simulink model "STModel_with_MMAE"  (R2018b)
settings: Solver=FixedStepDiscrete  StartTime=0.0  StopTime=6  FixedStep=Tsmall  RelTol=1e-3  EnableMultiTasking=on
PreLoadFcn:
  | if exist('tl_preloadfcn','file'), tl_preloadfcn(gcs,403); end
PostLoadFcn:
  | if exist('tl_postloadfcn','file'), tl_postloadfcn(gcs,403); end
InitFcn:
  | if exist('tlds_init','file'), tlds_init(gcs); end
StartFcn:
  | if exist('tlds_start','file'), tlds_start(gcs); end
StopFcn:
  | if exist('tlds_stop','file'), tlds_stop(gcs); end
values from neighbouring files (symbols this model uses):
  l = obj.vehicleParameters.l_r + obj.vehicleParameters.l_f    [SimplifiedKinematicBicycleModel.m]
  l_r = obj.vehicleParameters.l_r    [KinematicBicycleModel.m]
  Ts = 0.1    [KinematicBicycleModel.m]    (also in LeftLaneChangeSinusoidalMotionModel.m; LinearizedBicycleModel.m; SimplifiedKinematicBicycleModel.m; amm_rel_test.m)
  Ts_bp = 0.01    [initialization.m]    (also in laneChangeSinusoidalFcn.m; laneChangeSinusoidalJacobianFcn.m; leftLaneChangeParametricFcn.m; leftLaneChangeParametricWithAccFcn.m)
  vx = X(2)    [cv_model_fun.m]    (also in initialization.m = 10)
  vy = X(4)    [cv_model_fun.m]    (also in initialization.m = 0)
  x = X(1)    [KinematicBicycleModel.m]    (also in SimplifiedKinematicBicycleModel.m; behavior_model.m = 0:0.01:20; cca_model_fun.m; ctra_model_fun.m)
  y = X(2)    [KinematicBicycleModel.m]    (also in SimplifiedKinematicBicycleModel.m; behavior_model.m = [distances velocities]; cca_model_fun.m; ctra_model_fun.m)
undefined symbols (not defined in the file or in its folder): alpha_f0, alpha_r0, Bm1, Bsc, Bx_ash_f, Bx_ash_r, Bx_snow_f, Bx_snow_r, Bx_wash_f, Bx_wash_r, By_ash_f, By_ash_r, By_snow_f, By_snow_r, By_wash_f, By_wash_r, Cx_ash_f, Cx_ash_r, Cx_snow_f, Cx_snow_r, Cx_wash_f, Cx_wash_r, Cy_ash_f, Cy_ash_r, Cy_snow_f, Cy_snow_r, Cy_wash_f, Cy_wash_r, Ex_ash_f, Ex_ash_r, Ex_snow_f, Ex_snow_r, Ex_wash_f, Ex_wash_r, Ey_ash_f, Ey_ash_r, Ey_snow_f, Ey_snow_r, Ey_wash_f, Ey_wash_r, g, Im1, Isw, Iw, Iz, Kb1, Ks1, kt1, l_f, m, mu_x_ash_f, mu_x_ash_r, mu_x_snow_f, mu_x_snow_r, mu_x_wash_f, mu_x_wash_r, mu_y_ash_f, mu_y_ash_r, mu_y_snow_f, mu_y_snow_r ... (+18)
libraries: simulink x6
(part 1 of 2)
PreSaveFcn:
  | if exist('tl_presavefcn','file'), tl_presavefcn(gcs); end
CloseFcn:
  | if exist('tl_closefcn','file'), tl_closefcn(gcs); end
settings Model: TLRevision=403  ExtModeTrigDuration=10000  Creator=srivats  LastModifiedBy=jasprit
settings SolverCC: PositivePriorityOrder=on  AutoInsertRateTranBlk=on
settings DebuggingCC: LibraryContextMissingDiagnostic=none
settings SFSimCC: SimUseLocalCustomCode=off
settings RTWCC: SystemTargetFile=quarc_win64.tlc  TemplateMakefile=quarc_default_tmf  Description=QUARC Win64 Target  RTWUseLocalCustomCode=off
settings STFCustomTargetCC: TargetPreCompLibLocation=C:\PROGRA~3\QUARC\lib\2018a\win64\release  TargetLangStandard=C99 (ISO)  ConcurrentExecutionCompliant=on  GRTInterface=on  SystemTargetFile=quarc_win64.tlc
settings GRTTargetCC: TargetPreCompLibLocation=C:\PROGRA~3\QUARC\lib\2018a\win64\release  ParMdlRefBuildCompliant=off  CompOptLevelCompliant=off  CombineOutputUpdateFcns=off  MatFileLogging=off  CPPClassGenCompliant=off  GRTInterface=on  UseToolchainInfoCompliant=off  ExtMode=on  ExtModeMexFile=quarc_comm

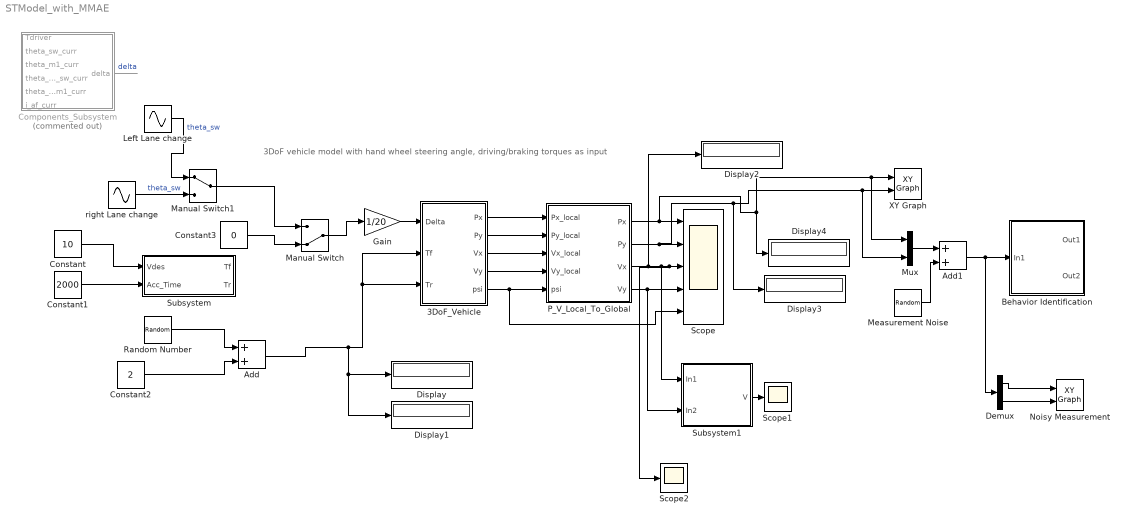
== system STModel_with_MMAE ==
  note: 3DoF vehicle model with hand wheel steering angle, driving/braking torques as input
  3DoF_Vehicle : Subsystem
  Add : Sum
  Add1 : Sum
  Behavior Identification : Subsystem
  Components_Subsystem : Subsystem  Commented=on
  Constant : Constant  Value=10
  Constant1 : Constant  Value=2000
  Constant2 : Constant  Value=2
  Constant3 : Constant  Value=0
  Demux : Demux  Outputs=2
  Display{,1..4} (5 alike) : Display
  Gain : Gain  Gain=1/20
  Left Lane change : Sin  Amplitude=0.11  Frequency=2*pi/10  SampleTime=0.001
  Manual Switch : ManualSwitch  CurrentSetting=0
  Manual Switch1 : ManualSwitch
  "Measurement Noise " : RandomNumber  Variance=0.025
  Mux : Mux  Inputs=2
  Noisy Measurement : simulink/Sinks/XY Graph  xmin=-10  xmax=100  ymin=-5  ymax=5  st=-1
  P_V_Local_To_Global : Subsystem
  Random Number : RandomNumber  SampleTime=0.001
  Scope : Scope  NumInputPorts=5
  Scope1 : Scope
  Scope2 : Scope
  Subsystem : Subsystem
  Subsystem1 : Subsystem
  XY Graph : simulink/Sinks/XY Graph  xmin=-10  xmax=100  ymin=-5  ymax=5  st=-1
  right Lane change : Sin  Amplitude=0.11  Frequency=2*pi/10  Phase=-pi  SampleTime=0.001
  wires:
  Components_Subsystem/1(delta) -> ?  "delta"
  3DoF_Vehicle/1(Px) -> P_V_Local_To_Global/1(Px_local)
  3DoF_Vehicle/2(Py) -> P_V_Local_To_Global/2(Py_local)
  3DoF_Vehicle/4(Vy) -> P_V_Local_To_Global/4(Vy_local)
  3DoF_Vehicle/5(psi) -> Scope/5, P_V_Local_To_Global/5(psi)
  P_V_Local_To_Global/1(Px) -> Display4/1, Mux/1, XY Graph/1, Scope/1
  P_V_Local_To_Global/2(Py) -> Display3/1, Mux/2, XY Graph/2, Scope/2
  P_V_Local_To_Global/3(Vx) -> Display2/1, Subsystem1/1(In1), Scope2/1, Scope/3
  P_V_Local_To_Global/4(Vy) -> Subsystem1/2(In2), Scope/4
  Gain/1 -> 3DoF_Vehicle/1(Delta)
  Left Lane change/1 -> Manual Switch1/1  "theta_sw"
  Constant/1 -> Subsystem/1(Vdes)
  Constant1/1 -> Subsystem/2(Acc_Time)
  Subsystem1/1(V) -> Scope1/1
  3DoF_Vehicle/3(Vx) -> P_V_Local_To_Global/3(Vx_local)
  Constant2/1 -> Add/2
  Add/1 -> Display1/1, Display/1, 3DoF_Vehicle/3(Tr), 3DoF_Vehicle/2(Tf)
  Random Number/1 -> Add/1
  Mux/1 -> Add1/1
  "Measurement Noise "/1 -> Add1/2
  Add1/1 -> Demux/1, Behavior Identification/1(In1)
  Demux/1 -> Noisy Measurement/1
  Demux/2 -> Noisy Measurement/2
  Constant3/1 -> Manual Switch/2
  Manual Switch/1 -> Gain/1
  Manual Switch1/1 -> Manual Switch/1
  right Lane change/1 -> Manual Switch1/2  "theta_sw"

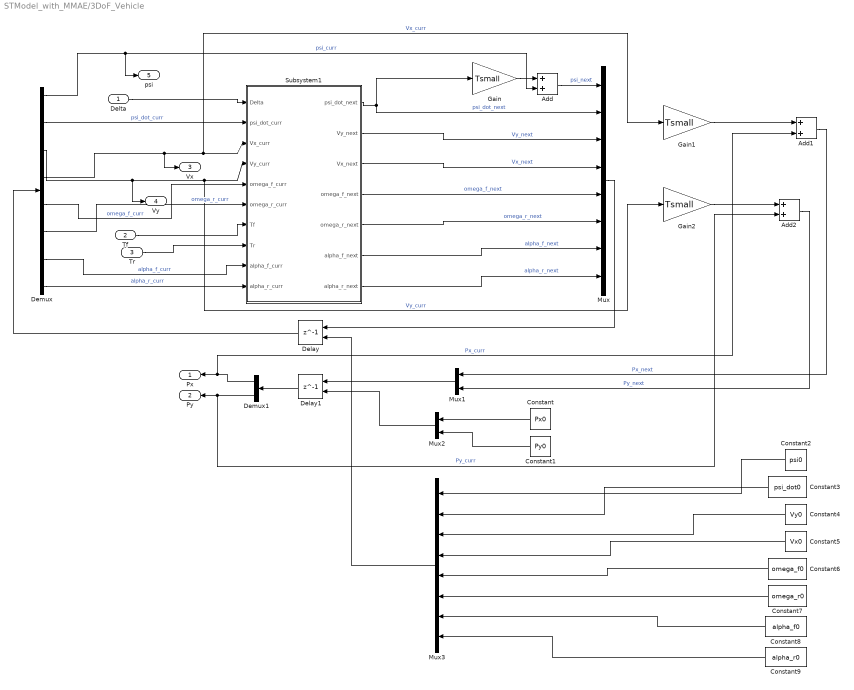
== system STModel_with_MMAE/3DoF_Vehicle ==
  Delta : Inport
  Tf : Inport  Port=2
  Tr : Inport  Port=3
  Add : Sum
  Add1 : Sum
  Add2 : Sum
  Constant : Constant  Value=Px0
  Constant1 : Constant  Value=Py0
  Constant2 : Constant  Value=psi0
  Constant3 : Constant  Value=psi_dot0
  Constant4 : Constant  Value=Vy0
  Constant5 : Constant  Value=Vx0
  Constant6 : Constant  Value=omega_f0
  Constant7 : Constant  Value=omega_r0
  Constant8 : Constant  Value=alpha_f0
  Constant9 : Constant  Value=alpha_r0
  Delay : Delay  DelayLength=1  InitialConditionSource=Input port  SampleTime=Tsmall
      settings: InputPortMap=u0,p4
  Delay1 : Delay  DelayLength=1  InitialConditionSource=Input port  SampleTime=Tsmall
      settings: InputPortMap=u0,p4
  Demux : Demux  Outputs=8
  Demux1 : Demux  Outputs=2
  Gain : Gain  Gain=Tsmall
  Gain1 : Gain  Gain=Tsmall
  Gain2 : Gain  Gain=Tsmall
  Mux : Mux  Inputs=8
  Mux1 : Mux  Inputs=2
  Mux2 : Mux  Inputs=2
  Mux3 : Mux  Inputs=8
  Subsystem1 : Subsystem
  Px : Outport
  Py : Outport  Port=2
  Vx : Outport  Port=3
  Vy : Outport  Port=4
  psi : Outport  Port=5
  wires:
  Demux/1 -> psi/1, Add/2  "psi_curr"
  Delay/1 -> Demux/1
  Demux/6 -> Subsystem1/6(omega_r_curr)  "omega_r_curr"
  Gain/1 -> Add/1
  Delta/1 -> Subsystem1/1(Delta)
  Subsystem1/4(omega_f_next) -> Mux/5  "omega_f_next"
  Subsystem1/1(psi_dot_next) -> Mux/2, Gain/1  "psi_dot_next"
  Add/1 -> Mux/1  "psi_next"
  Tr/1 -> Subsystem1/8(Tr)
  Tf/1 -> Subsystem1/7(Tf)
  Subsystem1/3(Vx_next) -> Mux/4  "Vx_next"
  Demux/2 -> Subsystem1/2(psi_dot_curr)  "psi_dot_curr"
  Mux/1 -> Delay/1
  Demux/4 -> Vx/1, Gain1/1, Subsystem1/3(Vx_curr)  "Vx_curr"
  Demux/3 -> Gain2/1, Subsystem1/4(Vy_curr), Vy/1  "Vy_curr"
  Demux/5 -> Subsystem1/5(omega_f_curr)  "omega_f_curr"
  Subsystem1/2(Vy_next) -> Mux/3  "Vy_next"
  Subsystem1/5(omega_r_next) -> Mux/6  "omega_r_next"
  Gain1/1 -> Add1/1
  Gain2/1 -> Add2/1
  Mux1/1 -> Delay1/1
  Add1/1 -> Mux1/1  "Px_next"
  Add2/1 -> Mux1/2  "Py_next"
  Mux2/1 -> Delay1/2
  Constant/1 -> Mux2/1
  Constant1/1 -> Mux2/2
  Delay1/1 -> Demux1/1
  Demux1/1 -> Add1/2, Px/1  "Px_curr"
  Demux1/2 -> Add2/2, Py/1  "Py_curr"
  Constant7/1 -> Mux3/6
  Constant6/1 -> Mux3/5
  Constant3/1 -> Mux3/2
  Constant5/1 -> Mux3/4
  Constant4/1 -> Mux3/3
  Constant2/1 -> Mux3/1
  Mux3/1 -> Delay/2
  Subsystem1/6(alpha_f_next) -> Mux/7  "alpha_f_next"
  Subsystem1/7(alpha_r_next) -> Mux/8  "alpha_r_next"
  Constant8/1 -> Mux3/7
  Constant9/1 -> Mux3/8
  Demux/7 -> Subsystem1/9(alpha_f_curr)  "alpha_f_curr"
  Demux/8 -> Subsystem1/10(alpha_r_curr)  "alpha_r_curr"

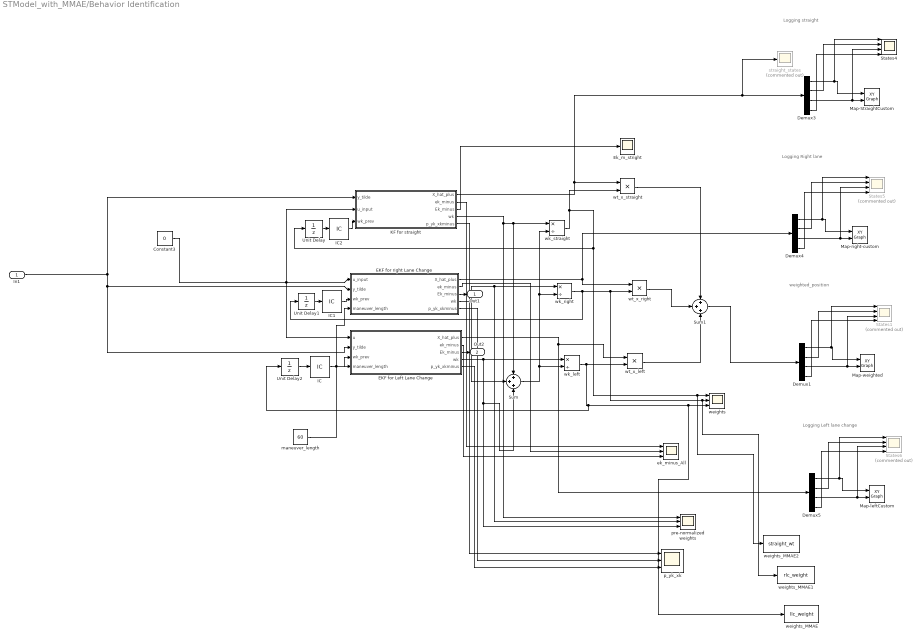
== system STModel_with_MMAE/Behavior Identification ==
  note: weighted_position
  note: Logging Right lane
  note: Logging straight
  note: Logging Left lane change
  In1 : Inport  SampleTime=Ts_bp
  Constant3 : Constant  Value=0
  Demux{1,3..5} (4 alike) : Demux
  EKF for Left Lane Change : Subsystem
  EKF for right Lane Change : Subsystem
  Ek_m_stright : Scope
  IC : InitialCondition  Value=1/3
  IC1 : InitialCondition  Value=1/3
  IC2 : InitialCondition  Value=1/3
  KF for straight : Subsystem
  Map-StraightCustom : simulink/Sinks/XY Graph  xmin=-1  xmax=200  ymin=-20  ymax=20  st=-1
  Map-leftCustom : simulink/Sinks/XY Graph  xmin=-1  xmax=300  ymin=-5  ymax=5  st=-1
  Map-right-custom : simulink/Sinks/XY Graph  xmin=-1  xmax=300  ymin=-5  ymax=5  st=-1
  Map-weighted : simulink/Sinks/XY Graph  xmin=-1  xmax=300  ymin=-5  ymax=5  st=-1
  States1 : Scope  Commented=on  NumInputPorts=4
  States4 : Scope  NumInputPorts=4
  States5 : Scope  Commented=on  NumInputPorts=4
  States6 : Scope  Commented=on  NumInputPorts=4
  Sum : Sum  Inputs=+++
  Sum1 : Sum  Inputs=+++
  Unit Delay : UnitDelay  SampleTime=Ts_bp
  Unit Delay1 : UnitDelay  SampleTime=Ts_bp
  Unit Delay2 : UnitDelay  SampleTime=Ts_bp
  ek_minus_All : Scope  NumInputPorts=3
  maneuver_length : Constant  Value=60
  p_yk_xk : Scope  NumInputPorts=3
  pre-normalized weights : Scope  NumInputPorts=3
  straight_states : Scope  Commented=on
  weights : Scope  NumInputPorts=3
  weights_MMAE : ToWorkspace  VariableName=llc_weight  SaveFormat=Structure With Time  SampleTime=-1
  weights_MMAE1 : ToWorkspace  VariableName=rlc_weight  SaveFormat=Structure With Time  SampleTime=-1
  weights_MMAE2 : ToWorkspace  VariableName=straight_wt  SaveFormat=Structure With Time  SampleTime=-1
  wk_left : Product  Inputs=*/
  wk_right : Product  Inputs=*/
  wk_straight : Product  Inputs=*/
  wt_x_left : Product  Inputs=**
  wt_x_right : Product  Inputs=**
  wt_x_straight : Product  Inputs=**
  Out1 : Outport
  Out2 : Outport  Port=2
  wires:
  Demux3/4 -> States4/4
  Demux1/2 -> States1/2
  EKF for Left Lane Change/2(ek_minus) -> ek_minus_All/3
  EKF for right Lane Change/1(X_hat_plus) -> Demux4/1, wt_x_right/1
  KF for straight/1(X_hat_plus) -> straight_states/1, Demux3/1, wt_x_straight/1
  In1/1 -> EKF for Left Lane Change/2(y_tilde), EKF for right Lane Change/2(y_tilde), KF for straight/1(y_tilde)
  wk_straight/1 -> Unit Delay/1, weights/1, weights_MMAE2/1, wt_x_straight/2
  wt_x_right/1 -> Sum1/2
  Demux4/3 -> Map-right-custom/2, States5/3
  EKF for Left Lane Change/1(X_hat_plus) -> wt_x_left/1, Demux5/1
  wk_left/1 -> Unit Delay2/1, weights_MMAE/1, weights/3, wt_x_left/2
  Demux5/1 -> States6/1, Map-leftCustom/1
  EKF for Left Lane Change/3(Ek_minus) -> Out2/1
  IC1/1 -> EKF for right Lane Change/3(wk_prev)
  maneuver_length/1 -> EKF for right Lane Change/4(maneuver_length), EKF for Left Lane Change/4(maneuver_length)
  EKF for right Lane Change/3(Ek_minus) -> Out1/1
  Demux1/1 -> States1/1, Map-weighted/1
  KF for straight/4(wk) -> pre-normalized weights/1, wk_straight/1, Sum/1
  KF for straight/5(p_yk_xkminus) -> p_yk_xk/1
  EKF for Left Lane Change/4(wk) -> wk_left/1, pre-normalized weights/3, Sum/3
  Sum/1 -> wk_left/2, wk_straight/2, wk_right/2
  Demux4/1 -> States5/1, Map-right-custom/1
  Demux1/4 -> States1/4
  Demux3/1 -> States4/1, Map-StraightCustom/1
  Constant3/1 -> KF for straight/2(u_input), EKF for right Lane Change/1(u_input), EKF for Left Lane Change/1(u)
  wk_right/1 -> Unit Delay1/1, weights_MMAE1/1, weights/2, wt_x_right/2
  Unit Delay/1 -> IC2/1
  wt_x_straight/1 -> Sum1/1
  EKF for right Lane Change/2(ek_minus) -> ek_minus_All/2
  Demux5/2 -> States6/2
  Demux5/3 -> Map-leftCustom/2, States6/3
  wt_x_left/1 -> Sum1/3
  Unit Delay2/1 -> IC/1
  Demux1/3 -> States1/3, Map-weighted/2
  KF for straight/2(ek_minus) -> ek_minus_All/1
  EKF for right Lane Change/4(wk) -> pre-normalized weights/2, wk_right/1, Sum/2
  EKF for Left Lane Change/5(p_yk_xkminus) -> p_yk_xk/3
  Demux5/4 -> States6/4
  Sum1/1 -> Demux1/1
  Unit Delay1/1 -> IC1/1
  Demux4/4 -> States5/4
  Demux3/3 -> Map-StraightCustom/2, States4/3
  EKF for right Lane Change/5(p_yk_xkminus) -> p_yk_xk/2
  IC/1 -> EKF for Left Lane Change/3(wk_prev)
  IC2/1 -> KF for straight/3(wk_prev)
  KF for straight/3(Ek_minus) -> Ek_m_stright/1
  Demux3/2 -> States4/2
  Demux4/2 -> States5/2

== system STModel_with_MMAE/Components_Subsystem ==
  Tdriver : Inport
  theta_sw_curr : Inport  Port=2
  theta_m1_curr : Inport  Port=3
  theta_dot_sw_curr : Inport  Port=4
  theta_dot_m1_curr : Inport  Port=5
  i_af_curr : Inport  Port=6
  Euler_Integrator1 : Subsystem
  Euler_Integrator2 : Subsystem
  Euler_Integrator3 : Subsystem
  Euler_Integrator4 : Subsystem
  Euler_Integrator5 : Subsystem
  Gain : Gain  Gain=kt1
  Subsystem : Subsystem
  Theta_M1_Subsystem : Subsystem
  Theta_SW_Subsystem : Subsystem
  delta : Outport
  wires:
  Tdriver/1 -> Theta_SW_Subsystem/1(Tdriver)
  theta_dot_sw_curr/1 -> Euler_Integrator1/1(state_dot), Euler_Integrator2/2(state_curr), Theta_SW_Subsystem/2(theta_dot_sw)
  theta_dot_m1_curr/1 -> Euler_Integrator4/1(state_dot), Euler_Integrator3/2(state_curr), Theta_SW_Subsystem/3(theta_dot_m1)  "theta_dot_m1"
  theta_sw_curr/1 -> Euler_Integrator1/2(state_curr), Theta_SW_Subsystem/4(theta_sw)
  theta_m1_curr/1 -> Euler_Integrator4/2(state_curr), Theta_SW_Subsystem/5(theta_m1)  "theta_m1_curr"
  Theta_SW_Subsystem/1(theta_sw_ddot) -> Euler_Integrator2/1(state_dot)
  Euler_Integrator2/1(state_next) -> ?  "theta_sw_dot_next"
  Euler_Integrator1/1(state_next) -> ?  "theta_sw_curr"
  Theta_M1_Subsystem/1("theta_m1_ddot ") -> Euler_Integrator3/1(state_dot)
  Euler_Integrator3/1(state_next) -> ?  "theta_m1_dot_next"
  Euler_Integrator4/1(state_next) -> ?  "theta_m1_next"
  i_af_curr/1 -> Gain/1, Euler_Integrator5/2(state_curr), Subsystem/1(i_a1)  "i_af"
  Subsystem/1(i_a1_dot) -> Euler_Integrator5/1(state_dot)
  Euler_Integrator5/1(state_next) -> ?  "i_af_next"
  Gain/1 -> Theta_M1_Subsystem/5(Tm1)

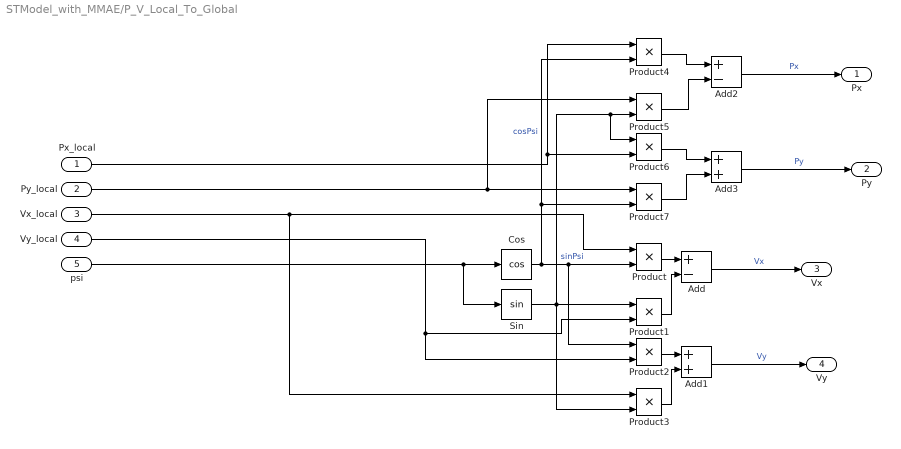
== system STModel_with_MMAE/P_V_Local_To_Global ==
  Px_local : Inport  OutDataTypeStr=double  SampleTime=Ts
  Py_local : Inport  Port=2  OutDataTypeStr=double  SampleTime=Ts
  Vx_local : Inport  Port=3  OutDataTypeStr=double  SampleTime=Ts
  Vy_local : Inport  Port=4  OutDataTypeStr=double  SampleTime=Ts
  psi : Inport  Port=5  OutDataTypeStr=double  SampleTime=Ts
  Add : Sum  Inputs=+-
  Add1 : Sum
  Add2 : Sum  Inputs=+-
  Add3 : Sum
  Cos : Trigonometry  Operator=cos
  Product{,1..7} (8 alike) : Product
  Sin : Trigonometry
  Px : Outport  OutDataTypeStr=double  SampleTime=Ts
  Py : Outport  Port=2  OutDataTypeStr=double  SampleTime=Ts
  Vx : Outport  Port=3  OutDataTypeStr=double  SampleTime=Ts
  Vy : Outport  Port=4  OutDataTypeStr=double  SampleTime=Ts
  wires:
  Px_local/1 -> Product4/1, Product6/2
  Py_local/1 -> Product7/1, Product5/1
  Vx_local/1 -> Product3/1, Product/1
  Product5/1 -> Add2/2
  Product4/1 -> Add2/1
  Add2/1 -> Px/1  "Px"
  Product7/1 -> Add3/2
  Sin/1 -> Product6/1, Product5/2, Product3/2, Product1/1  "sinPsi"
  Vy_local/1 -> Product1/2, Product2/2
  psi/1 -> Sin/1, Cos/1
  Cos/1 -> Product7/2, Product4/2, Product2/1, Product/2  "cosPsi"
  Add3/1 -> Py/1  "Py"
  Product2/1 -> Add1/1
  Product1/1 -> Add/2
  Add/1 -> Vx/1  "Vx"
  Add1/1 -> Vy/1  "Vy"
  Product6/1 -> Add3/1
  Product3/1 -> Add1/2
  Product/1 -> Add/1

== system STModel_with_MMAE/Subsystem ==
  Vdes : Inport
  Acc_Time : Inport  Port=2
  Add : Sum
  Constant : Constant  Value=RR
  Divide : Product  Inputs=*/
  Gain : Gain  Gain=9.81
  Gain1 : Gain  Gain=m
  Gain2 : Gain  Gain=0.5
  Tf : Outport
  Tr : Outport  Port=2
  wires:
  Vdes/1 -> Gain1/1
  Acc_Time/1 -> Gain/1
  Gain1/1 -> Divide/1
  Gain/1 -> Divide/2
  Divide/1 -> Add/1  "Fa"
  Constant/1 -> Add/2
  Add/1 -> Gain2/1  "TTE"
  Gain2/1 -> Tf/1, Tr/1

== system STModel_with_MMAE/Subsystem1 ==
  In1 : Inport
  In2 : Inport  Port=2
  Add : Sum
  Sqrt : Sqrt  SaturateOnIntegerOverflow=on
  Square : Math  Operator=square  SaturateOnIntegerOverflow=on
  Square1 : Math  Operator=square  SaturateOnIntegerOverflow=on
  V : Outport
  wires:
  Square1/1 -> Add/2
  In1/1 -> Square/1
  Add/1 -> Sqrt/1
  Square/1 -> Add/1
  Sqrt/1 -> V/1  "V"
  In2/1 -> Square1/1

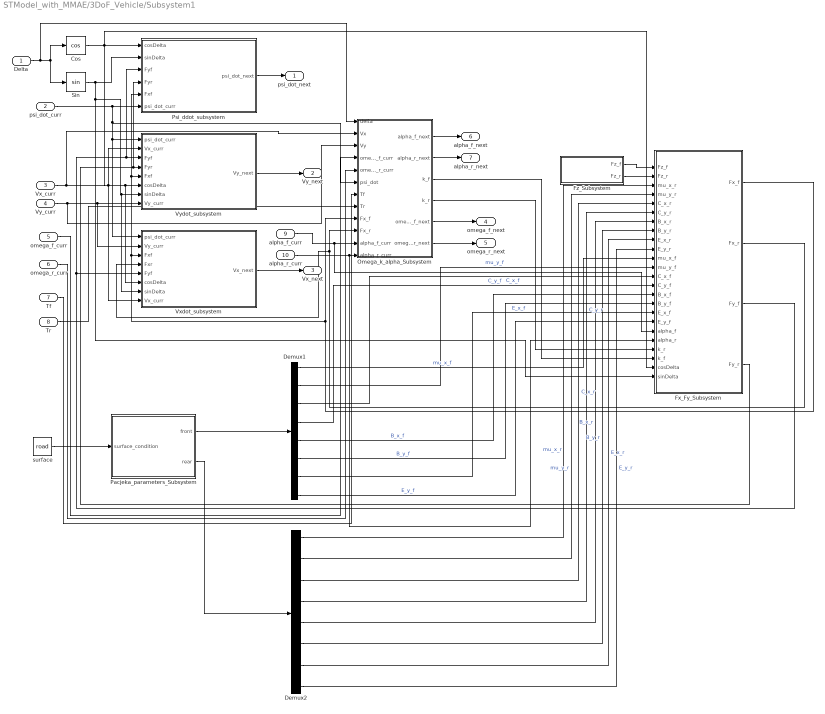
== system STModel_with_MMAE/3DoF_Vehicle/Subsystem1 ==
  Delta : Inport
  psi_dot_curr : Inport  Port=2
  Vx_curr : Inport  Port=3
  Vy_curr : Inport  Port=4
  omega_f_curr : Inport  Port=5
  omega_r_curr : Inport  Port=6
  Tf : Inport  Port=7
  Tr : Inport  Port=8
  alpha_f_curr : Inport  Port=9
  alpha_r_curr : Inport  Port=10
  Cos : Trigonometry  Operator=cos
  Demux1 : Demux  Outputs=8
  Demux2 : Demux  Outputs=8
  Fx_Fy_Subsystem : Subsystem
  Fz_Subsystem : Subsystem
  Omega_k_alpha_Subsystem : Subsystem
  Pacjeka_parameters_Subsystem : Subsystem
  Psi_ddot_subsystem : Subsystem
  Sin : Trigonometry
  Vxdot_subsystem : Subsystem
  Vydot_subsystem : Subsystem
  surface : Constant  Value=road
  psi_dot_next : Outport
  Vy_next : Outport  Port=2
  Vx_next : Outport  Port=3
  omega_f_next : Outport  Port=4
  omega_r_next : Outport  Port=5
  alpha_f_next : Outport  Port=6
  alpha_r_next : Outport  Port=7
  wires:
  Omega_k_alpha_Subsystem/4(k_r) -> Fx_Fy_Subsystem/21(k_r)
  Fx_Fy_Subsystem/2(Fx_r) -> Vxdot_subsystem/4(Fxr), Omega_k_alpha_Subsystem/10(Fx_r)
  Fx_Fy_Subsystem/1(Fx_f) -> Omega_k_alpha_Subsystem/9(Fx_f), Vxdot_subsystem/3(Fxf), Psi_ddot_subsystem/5(Fxf), Vydot_subsystem/5(Fxf)
  Omega_k_alpha_Subsystem/3(k_f) -> Fx_Fy_Subsystem/22(k_f)
  Sin/1 -> Fx_Fy_Subsystem/24(sinDelta), Vxdot_subsystem/7(sinDelta), Vydot_subsystem/7(sinDelta), Psi_ddot_subsystem/2(sinDelta)
  Vydot_subsystem/1(Vy_next) -> Vy_next/1
  Fx_Fy_Subsystem/3(Fy_f) -> Psi_ddot_subsystem/3(Fyf), Vydot_subsystem/3(Fyf), Vxdot_subsystem/5(Fyf)
  psi_dot_curr/1 -> Omega_k_alpha_Subsystem/6(psi_dot), Vydot_subsystem/1(psi_dot_curr), Vxdot_subsystem/1(psi_dot_curr), Psi_ddot_subsystem/6(psi_dot_curr)
  Fx_Fy_Subsystem/4(Fy_r) -> Psi_ddot_subsystem/4(Fyr), Vydot_subsystem/4(Fyr)
  Cos/1 -> Fx_Fy_Subsystem/23(cosDelta), Vxdot_subsystem/6(cosDelta), Vydot_subsystem/6(cosDelta), Psi_ddot_subsystem/1(cosDelta)
  Tf/1 -> Omega_k_alpha_Subsystem/7(Tf)
  Demux1/7 -> Fx_Fy_Subsystem/17(E_x_f)  "E_x_f"
  omega_f_curr/1 -> Omega_k_alpha_Subsystem/4(omega_f_curr)
  Vy_curr/1 -> Omega_k_alpha_Subsystem/3(Vy), Vxdot_subsystem/2(Vy_curr), Vydot_subsystem/8(Vy_curr)
  Pacjeka_parameters_Subsystem/1(front) -> Demux1/1
  Omega_k_alpha_Subsystem/6(omega_r_next) -> omega_r_next/1
  Delta/1 -> Omega_k_alpha_Subsystem/1(delta), Sin/1, Cos/1
  Vx_curr/1 -> Omega_k_alpha_Subsystem/2(Vx), Vydot_subsystem/2(Vx_curr), Vxdot_subsystem/8(Vx_curr)
  Demux1/1 -> Fx_Fy_Subsystem/11(mu_x_f)  "mu_x_f"
  Vxdot_subsystem/1(Vx_next) -> Vx_next/1
  Omega_k_alpha_Subsystem/5(omega_f_next) -> omega_f_next/1
  Demux2/4 -> Fx_Fy_Subsystem/6(C_y_r)  "C_y_r"
  Fz_Subsystem/1(Fz_f) -> Fx_Fy_Subsystem/1(Fz_f)
  Tr/1 -> Omega_k_alpha_Subsystem/8(Tr)
  omega_r_curr/1 -> Omega_k_alpha_Subsystem/5(omega_r_curr)
  surface/1 -> Pacjeka_parameters_Subsystem/1(surface_condition)
  Pacjeka_parameters_Subsystem/2(rear) -> Demux2/1
  Demux2/7 -> Fx_Fy_Subsystem/9(E_x_r)  "E_x_r"
  Fz_Subsystem/2(Fz_r) -> Fx_Fy_Subsystem/2(Fz_r)
  Demux1/6 -> Fx_Fy_Subsystem/16(B_y_f)  "B_y_f"
  Demux2/6 -> Fx_Fy_Subsystem/8(B_y_r)  "B_y_r"
  Demux2/2 -> Fx_Fy_Subsystem/4(mu_y_r)  "mu_y_r"
  Demux1/8 -> Fx_Fy_Subsystem/18(E_y_f)  "E_y_f"
  Demux2/5 -> Fx_Fy_Subsystem/7(B_x_r)  "B_x_r"
  Psi_ddot_subsystem/1(psi_dot_next) -> psi_dot_next/1
  Demux2/8 -> Fx_Fy_Subsystem/10(E_y_r)  "E_y_r"
  Demux2/1 -> Fx_Fy_Subsystem/3(mu_x_r)  "mu_x_r"
  Demux1/3 -> Fx_Fy_Subsystem/13(C_x_f)  "C_x_f"
  Demux1/4 -> Fx_Fy_Subsystem/14(C_y_f)  "C_y_f"
  Demux1/2 -> Fx_Fy_Subsystem/12(mu_y_f)  "mu_y_f"
  Demux1/5 -> Fx_Fy_Subsystem/15(B_x_f)  "B_x_f"
  Demux2/3 -> Fx_Fy_Subsystem/5(C_x_r)  "C_x_r"
  Omega_k_alpha_Subsystem/1(alpha_f_next) -> alpha_f_next/1
  Omega_k_alpha_Subsystem/2(alpha_r_next) -> alpha_r_next/1
  alpha_r_curr/1 -> Fx_Fy_Subsystem/20(alpha_r), Omega_k_alpha_Subsystem/12(alpha_r_curr)
  alpha_f_curr/1 -> Fx_Fy_Subsystem/19(alpha_f), Omega_k_alpha_Subsystem/11(alpha_f_curr)

== system STModel_with_MMAE/Behavior Identification/EKF for Left Lane Change ==
  u : Inport
  y_tilde : Inport  Port=2
  wk_prev : Inport  Port=3
  maneuver_length : Inport  Port=4
  IC3 : InitialCondition  Value=[x vx y vy]
  MATLAB Function2 : MATLAB Function  TreatAsAtomicUnit=on
  Unit Delay5 : UnitDelay  SampleTime=-1
  Unit Delay6 : UnitDelay  InitialCondition=eye(4)*100  SampleTime=-1
  X_hat_plus : Outport
  ek_minus : Outport  Port=2
  Ek_minus : Outport  Port=3
  wk : Outport  Port=4
  p_yk_xkminus : Outport  Port=5
  wires:
  MATLAB Function2/2(P_plus) -> Unit Delay6/1
  u/1 -> MATLAB Function2/3(u)
  Unit Delay5/1 -> IC3/1
  y_tilde/1 -> MATLAB Function2/4(y_tilde)
  MATLAB Function2/1(X_hat_plus) -> X_hat_plus/1, Unit Delay5/1
  IC3/1 -> MATLAB Function2/1(X)
  Unit Delay6/1 -> MATLAB Function2/2(P)
  MATLAB Function2/3(ek_minus) -> ek_minus/1
  MATLAB Function2/4(ek_m_covariance) -> Ek_minus/1
  MATLAB Function2/5(wk) -> wk/1
  MATLAB Function2/6(p_yk_xkminus) -> p_yk_xkminus/1
  wk_prev/1 -> MATLAB Function2/5(wk_prev)
  maneuver_length/1 -> MATLAB Function2/6(maneuver_length)

== system STModel_with_MMAE/Behavior Identification/EKF for right Lane Change ==
  note: Prior - right lane change
  u_input : Inport
  y_tilde : Inport  Port=2
  wk_prev : Inport  Port=3
  maneuver_length : Inport  Port=4
  IC2 : InitialCondition  Value=[x vx y vy]
  MATLAB Function1 : MATLAB Function  TreatAsAtomicUnit=on
  Unit Delay3 : UnitDelay  InitialCondition=eye(4)*100  SampleTime=-1
  Unit Delay4 : UnitDelay  SampleTime=-1
  X_hat_plus : Outport
  ek_minus : Outport  Port=2
  Ek_minus : Outport  Port=3
  wk : Outport  Port=4
  p_yk_xkminus : Outport  Port=5
  wires:
  MATLAB Function1/2(P_plus) -> Unit Delay3/1
  IC2/1 -> MATLAB Function1/1(X)
  Unit Delay3/1 -> MATLAB Function1/2(P)
  MATLAB Function1/1(X_hat_plus) -> X_hat_plus/1, Unit Delay4/1
  u_input/1 -> MATLAB Function1/3(u)
  y_tilde/1 -> MATLAB Function1/4(y_tilde)
  Unit Delay4/1 -> IC2/1
  MATLAB Function1/3(ek_minus) -> ek_minus/1
  MATLAB Function1/4(ek_m_covariance) -> Ek_minus/1
  wk_prev/1 -> MATLAB Function1/5(wk_prev)
  MATLAB Function1/5(wk) -> wk/1
  MATLAB Function1/6(p_yk_xkminus) -> p_yk_xkminus/1
  maneuver_length/1 -> MATLAB Function1/6(maneuver_length)

== system STModel_with_MMAE/Behavior Identification/KF for straight ==
  note: Prior
  y_tilde : Inport
  u_input : Inport  Port=2
  wk_prev : Inport  Port=3
  IC1 : InitialCondition  Value=[x vx y vy]
  MATLAB Function : MATLAB Function  TreatAsAtomicUnit=on
  Scope : Scope
  Scope1 : Scope
  Unit Delay1 : UnitDelay  SampleTime=-1
  Unit Delay2 : UnitDelay  InitialCondition=eye(4)*100  SampleTime=-1
  X_hat_plus : Outport
  ek_minus : Outport  Port=2
  Ek_minus : Outport  Port=3
  wk : Outport  Port=4
  p_yk_xkminus : Outport  Port=5
  wires:
  Unit Delay2/1 -> MATLAB Function/2(P)
  IC1/1 -> MATLAB Function/1(X)
  MATLAB Function/1(X_hat_plus) -> X_hat_plus/1, Unit Delay1/1
  u_input/1 -> MATLAB Function/3(u)
  Unit Delay1/1 -> IC1/1
  y_tilde/1 -> MATLAB Function/4(y_tilde)
  MATLAB Function/2(P_plus) -> Scope/1, Unit Delay2/1
  MATLAB Function/3(ek_minus) -> ek_minus/1
  MATLAB Function/4(ek_m_covariance) -> Ek_minus/1
  wk_prev/1 -> MATLAB Function/5(wk_prev)
  MATLAB Function/5(wk) -> wk/1
  MATLAB Function/6(p_yk_xkminus) -> p_yk_xkminus/1
  MATLAB Function/7(K) -> Scope1/1

== system STModel_with_MMAE/Components_Subsystem/Euler_Integrator1 ==
  state_dot : Inport
  state_curr : Inport  Port=2
  Add : Sum
  Gain : Gain  Gain=Tsmall
  state_next : Outport
  wires:
  state_dot/1 -> Gain/1
  Gain/1 -> Add/1
  state_curr/1 -> Add/2
  Add/1 -> state_next/1

== system STModel_with_MMAE/Components_Subsystem/Euler_Integrator2 ==
  state_dot : Inport
  state_curr : Inport  Port=2
  Add : Sum
  Gain : Gain  Gain=Tsmall
  state_next : Outport
  wires:
  state_dot/1 -> Gain/1
  Gain/1 -> Add/1
  state_curr/1 -> Add/2
  Add/1 -> state_next/1

== system STModel_with_MMAE/Components_Subsystem/Euler_Integrator3 ==
  state_dot : Inport
  state_curr : Inport  Port=2
  Add : Sum
  Gain : Gain  Gain=Tsmall
  state_next : Outport
  wires:
  state_dot/1 -> Gain/1
  Gain/1 -> Add/1
  state_curr/1 -> Add/2
  Add/1 -> state_next/1

== system STModel_with_MMAE/Components_Subsystem/Euler_Integrator4 ==
  state_dot : Inport
  state_curr : Inport  Port=2
  Add : Sum
  Gain : Gain  Gain=Tsmall
  state_next : Outport
  wires:
  state_dot/1 -> Gain/1
  Gain/1 -> Add/1
  state_curr/1 -> Add/2
  Add/1 -> state_next/1

== system STModel_with_MMAE/Components_Subsystem/Euler_Integrator5 ==
  state_dot : Inport
  state_curr : Inport  Port=2
  Add : Sum
  Gain : Gain  Gain=Tsmall
  state_next : Outport
  wires:
  state_dot/1 -> Gain/1
  Gain/1 -> Add/1
  state_curr/1 -> Add/2
  Add/1 -> state_next/1

== system STModel_with_MMAE/Components_Subsystem/Subsystem ==
  i_a1 : Inport
  theta_dot_M1 : Inport  Port=2
  Vs1 : Inport  Port=3
  Add : Sum  Inputs=--+
  Gain : Gain  Gain=R1
  Gain1 : Gain  Gain=Kb1
  i_a1_dot : Outport
  wires:
  Gain/1 -> Add/1
  Gain1/1 -> Add/2
  i_a1/1 -> Gain/1
  theta_dot_M1/1 -> Gain1/1
  Vs1/1 -> Add/3

== system STModel_with_MMAE/Components_Subsystem/Theta_M1_Subsystem ==
  theta_dot_sw : Inport
  theta_dot_m1 : Inport  Port=2
  theta_sw : Inport  Port=3
  theta_m1 : Inport  Port=4
  Tm1 : Inport  Port=5
  Add : Sum  Inputs=---+
  Gain : Gain  Gain=Bsc
  Gain1 : Gain  Gain=Ks1
  Gain2 : Gain  Gain=Bm1
  Gain3 : Gain  Gain=1/Im1
  Subtract : Sum  Inputs=+-
  Subtract1 : Sum  Inputs=+-
  "theta_m1_ddot " : Outport
  wires:
  theta_m1/1 -> Subtract/1
  theta_sw/1 -> Subtract/2
  theta_dot_m1/1 -> Gain2/1, Subtract1/1
  theta_dot_sw/1 -> Subtract1/2
  Subtract/1 -> Gain1/1
  Subtract1/1 -> Gain/1
  Gain/1 -> Add/1
  Gain1/1 -> Add/3
  Gain2/1 -> Add/2
  Tm1/1 -> Add/4
  Add/1 -> Gain3/1
  Gain3/1 -> "theta_m1_ddot "/1

== system STModel_with_MMAE/Components_Subsystem/Theta_SW_Subsystem ==
  Tdriver : Inport
  theta_dot_sw : Inport  Port=2
  theta_dot_m1 : Inport  Port=3
  theta_sw : Inport  Port=4
  theta_m1 : Inport  Port=5
  Constant : Constant  Value=Tfr_c
  Gain : Gain  Gain=Bsc
  Gain1 : Gain  Gain=Ks1
  Gain2 : Gain  Gain=1/Isw
  Subtract : Sum  Inputs=+-
  Subtract1 : Sum  Inputs=+---
  Subtract2 : Sum  Inputs=+-
  theta_sw_ddot : Outport
  wires:
  Subtract/1 -> Gain/1
  Constant/1 -> Subtract1/4
  theta_m1/1 -> Subtract2/2
  theta_sw/1 -> Subtract2/1
  Gain/1 -> Subtract1/2
  theta_dot_m1/1 -> Subtract/2
  theta_dot_sw/1 -> Subtract/1
  Subtract1/1 -> Gain2/1
  Gain1/1 -> Subtract1/3
  Subtract2/1 -> Gain1/1
  Tdriver/1 -> Subtract1/1
  Gain2/1 -> theta_sw_ddot/1

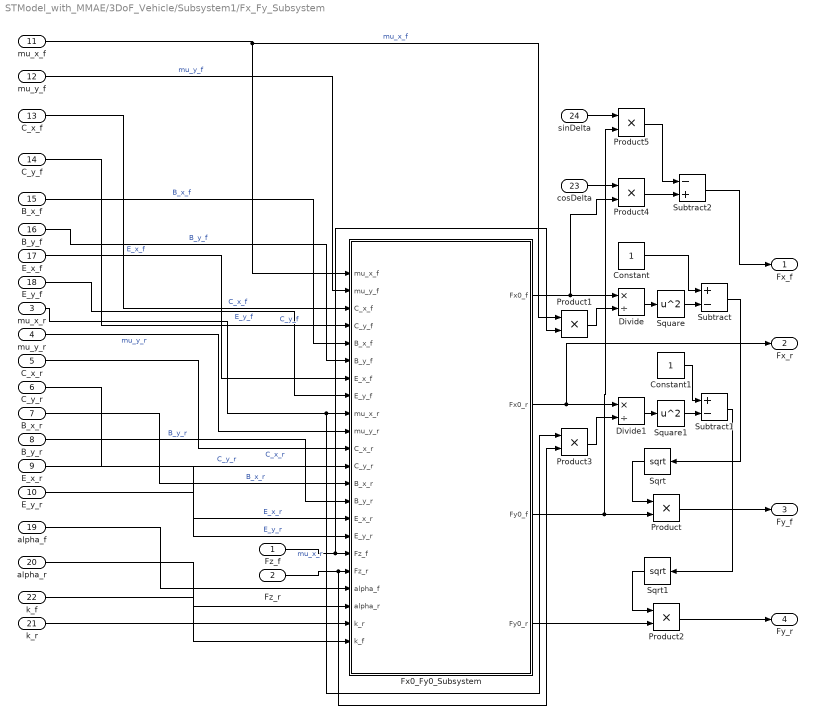
== system STModel_with_MMAE/3DoF_Vehicle/Subsystem1/Fx_Fy_Subsystem ==
  Fz_f : Inport
  Fz_r : Inport  Port=2
  mu_x_r : Inport  Port=3
  mu_y_r : Inport  Port=4
  C_x_r : Inport  Port=5
  C_y_r : Inport  Port=6
  B_x_r : Inport  Port=7
  B_y_r : Inport  Port=8
  E_x_r : Inport  Port=9
  E_y_r : Inport  Port=10
  mu_x_f : Inport  Port=11
  mu_y_f : Inport  Port=12
  C_x_f : Inport  Port=13
  C_y_f : Inport  Port=14
  B_x_f : Inport  Port=15
  B_y_f : Inport  Port=16
  E_x_f : Inport  Port=17
  E_y_f : Inport  Port=18
  alpha_f : Inport  Port=19
  alpha_r : Inport  Port=20
  k_r : Inport  Port=21
  k_f : Inport  Port=22
  cosDelta : Inport  Port=23
  sinDelta : Inport  Port=24
  Constant : Constant
  Constant1 : Constant
  Divide : Product  Inputs=*/
  Divide1 : Product  Inputs=*/
  Fx0_Fy0_Subsystem : Subsystem
  Product{,1..5} (6 alike) : Product
  Sqrt : Sqrt  SaturateOnIntegerOverflow=on
  Sqrt1 : Sqrt  SaturateOnIntegerOverflow=on
  Square : Math  Operator=square  SaturateOnIntegerOverflow=on
  Square1 : Math  Operator=square  SaturateOnIntegerOverflow=on
  Subtract : Sum  Inputs=+-
  Subtract1 : Sum  Inputs=+-
  Subtract2 : Sum  Inputs=-+
  Fx_f : Outport
  Fx_r : Outport  Port=2
  Fy_f : Outport  Port=3
  Fy_r : Outport  Port=4
  wires:
  B_x_r/1 -> Fx0_Fy0_Subsystem/13(B_x_r)  "B_x_r"
  mu_y_r/1 -> Fx0_Fy0_Subsystem/10(mu_y_r)  "mu_y_r"
  C_x_r/1 -> Fx0_Fy0_Subsystem/11(C_x_r)  "C_x_r"
  E_y_r/1 -> Fx0_Fy0_Subsystem/16(E_y_r)  "E_y_r"
  mu_x_r/1 -> Fx0_Fy0_Subsystem/9(mu_x_r), Product3/1  "mu_x_r"
  C_y_r/1 -> Fx0_Fy0_Subsystem/12(C_y_r)  "C_y_r"
  E_x_r/1 -> Fx0_Fy0_Subsystem/15(E_x_r)  "E_x_r"
  B_y_r/1 -> Fx0_Fy0_Subsystem/14(B_y_r)  "B_y_r"
  B_x_f/1 -> Fx0_Fy0_Subsystem/5(B_x_f)  "B_x_f"
  mu_y_f/1 -> Fx0_Fy0_Subsystem/2(mu_y_f)  "mu_y_f"
  C_x_f/1 -> Fx0_Fy0_Subsystem/3(C_x_f)  "C_x_f"
  E_y_f/1 -> Fx0_Fy0_Subsystem/8(E_y_f)  "E_y_f"
  mu_x_f/1 -> Product1/1, Fx0_Fy0_Subsystem/1(mu_x_f)  "mu_x_f"
  C_y_f/1 -> Fx0_Fy0_Subsystem/4(C_y_f)  "C_y_f"
  E_x_f/1 -> Fx0_Fy0_Subsystem/7(E_x_f)  "E_x_f"
  B_y_f/1 -> Fx0_Fy0_Subsystem/6(B_y_f)  "B_y_f"
  Fz_f/1 -> Product1/2, Fx0_Fy0_Subsystem/17(Fz_f)
  Fz_r/1 -> Product3/2, Fx0_Fy0_Subsystem/18(Fz_r)
  alpha_f/1 -> Fx0_Fy0_Subsystem/19(alpha_f)
  alpha_r/1 -> Fx0_Fy0_Subsystem/20(alpha_r)
  k_f/1 -> Fx0_Fy0_Subsystem/22(k_f)
  k_r/1 -> Fx0_Fy0_Subsystem/21(k_r)
  Constant/1 -> Subtract/1
  Fx0_Fy0_Subsystem/1(Fx0_f) -> Product4/2, Divide/1
  Product1/1 -> Divide/2
  Divide/1 -> Square/1
  Subtract/1 -> Sqrt/1
  Square/1 -> Subtract/2
  Sqrt/1 -> Product/1
  Product/1 -> Fy_f/1
  Product2/1 -> Fy_r/1
  Fx0_Fy0_Subsystem/4(Fy0_r) -> Product2/2
  Sqrt1/1 -> Product2/1
  Divide1/1 -> Square1/1
  Square1/1 -> Subtract1/2
  Product3/1 -> Divide1/2
  Fx0_Fy0_Subsystem/2(Fx0_r) -> Fx_r/1, Divide1/1
  Constant1/1 -> Subtract1/1
  Subtract1/1 -> Sqrt1/1
  cosDelta/1 -> Product4/1
  Product4/1 -> Subtract2/2
  sinDelta/1 -> Product5/1
  Fx0_Fy0_Subsystem/3(Fy0_f) -> Product5/2, Product/2
  Product5/1 -> Subtract2/1
  Subtract2/1 -> Fx_f/1

== system STModel_with_MMAE/3DoF_Vehicle/Subsystem1/Fz_Subsystem ==
  Constant : Constant  Value=(m*g*l_f)/l
  Constant1 : Constant  Value=(m*g*l_r)/l
  Fz_f : Outport
  Fz_r : Outport  Port=2
  wires:
  Constant/1 -> Fz_r/1
  Constant1/1 -> Fz_f/1

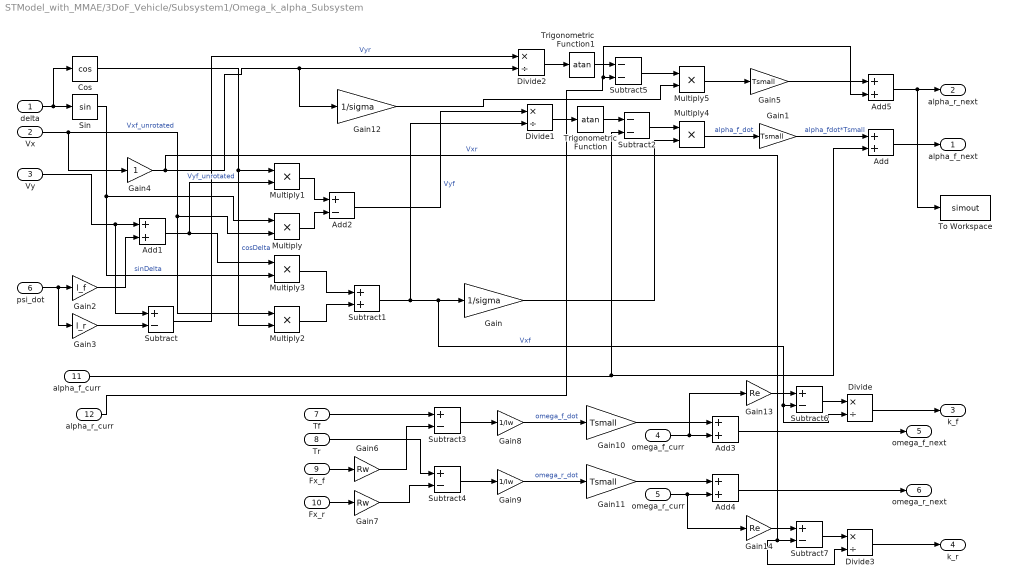
== system STModel_with_MMAE/3DoF_Vehicle/Subsystem1/Omega_k_alpha_Subsystem ==
  delta : Inport
  Vx : Inport  Port=2
  Vy : Inport  Port=3
  omega_f_curr : Inport  Port=4
  omega_r_curr : Inport  Port=5
  psi_dot : Inport  Port=6
  Tf : Inport  Port=7
  Tr : Inport  Port=8
  Fx_f : Inport  Port=9
  Fx_r : Inport  Port=10
  alpha_f_curr : Inport  Port=11
  alpha_r_curr : Inport  Port=12
  Add{,1,3..5} (5 alike) : Sum
  Add2 : Sum  Inputs=+-
  Cos : Trigonometry  Operator=cos
  Divide{,1..3} (4 alike) : Product  Inputs=*/
  Gain : Gain  Gain=1/sigma
  Gain{1,5,10..11} (4 alike) : Gain  Gain=Tsmall
  Gain12 : Gain  Gain=1/sigma
  Gain13 : Gain  Gain=Re
  Gain14 : Gain  Gain=Re
  Gain2 : Gain  Gain=l_f
  Gain3 : Gain  Gain=l_r
  Gain4 : Gain
  Gain6 : Gain  Gain=Rw
  Gain7 : Gain  Gain=Rw
  Gain8 : Gain  Gain=1/Iw
  Gain9 : Gain  Gain=1/Iw
  Multiply{,1..5} (6 alike) : Product
  Sin : Trigonometry
  Subtract{,3..4,6..7} (5 alike) : Sum  Inputs=+-
  Subtract1 : Sum
  Subtract2 : Sum  Inputs=--
  Subtract5 : Sum  Inputs=--
  To Workspace : ToWorkspace  VariableName=simout  SaveFormat=Timeseries  SampleTime=-1
  Trigonometric Function : Trigonometry  Operator=atan
  Trigonometric Function1 : Trigonometry  Operator=atan
  alpha_f_next : Outport
  alpha_r_next : Outport  Port=2
  k_f : Outport  Port=3
  k_r : Outport  Port=4
  omega_f_next : Outport  Port=5
  omega_r_next : Outport  Port=6
  wires:
  Fx_f/1 -> Gain6/1
  Fx_r/1 -> Gain7/1
  Tf/1 -> Subtract3/1
  Gain6/1 -> Subtract3/2
  Tr/1 -> Subtract4/1
  Gain7/1 -> Subtract4/2
  Subtract3/1 -> Gain8/1
  Subtract4/1 -> Gain9/1
  Gain8/1 -> Gain10/1  "omega_f_dot"
  Gain9/1 -> Gain11/1  "omega_r_dot"
  Gain10/1 -> Add3/1
  Gain11/1 -> Add4/1
  Add3/1 -> omega_f_next/1
  Add4/1 -> omega_r_next/1
  omega_f_curr/1 -> Gain13/1, Add3/2
  Multiply4/1 -> Gain1/1  "alpha_f_dot"
  Gain1/1 -> Add/1  "alpha_fdot*Tsmall"
  Divide1/1 -> Trigonometric Function/1
  omega_r_curr/1 -> Gain14/1, Add4/2
  psi_dot/1 -> Gain3/1, Gain2/1
  Gain2/1 -> Add1/2
  Vy/1 -> Subtract/1, Add1/1
  Add1/1 -> Multiply1/2, Multiply3/1  "Vyf_unrotated"
  Gain3/1 -> Subtract/2
  Subtract/1 -> Divide2/1  "Vyr"
  Vx/1 -> Multiply/2, Multiply2/1, Gain4/1  "Vxf_unrotated"
  Gain4/1 -> Subtract7/2, Divide3/2, Gain12/1, Divide2/2  "Vxr"
  delta/1 -> Cos/1, Sin/1
  Cos/1 -> Multiply2/2, Multiply1/1  "cosDelta"
  Multiply1/1 -> Add2/1
  Multiply/1 -> Add2/2
  Add2/1 -> Divide1/1  "Vyf"
  Multiply3/1 -> Subtract1/1
  Multiply2/1 -> Subtract1/2
  Subtract1/1 -> Divide/2, Subtract6/2, Gain/1, Divide1/2  "Vxf"
  Trigonometric Function/1 -> Subtract2/1
  alpha_f_curr/1 -> Add/2, Subtract2/2
  Subtract2/1 -> Multiply4/1
  Gain/1 -> Multiply4/2
  Add/1 -> alpha_f_next/1
  Subtract5/1 -> Multiply5/1
  Trigonometric Function1/1 -> Subtract5/1
  Divide2/1 -> Trigonometric Function1/1
  Multiply5/1 -> Gain5/1
  Gain5/1 -> Add5/1
  Add5/1 -> To Workspace/1, alpha_r_next/1
  alpha_r_curr/1 -> Add5/2, Subtract5/2
  Gain12/1 -> Multiply5/2
  Gain13/1 -> Subtract6/1
  Subtract6/1 -> Divide/1
  Divide/1 -> k_f/1
  Gain14/1 -> Subtract7/1
  Subtract7/1 -> Divide3/1
  Divide3/1 -> k_r/1
  Sin/1 -> Multiply/1, Multiply3/2  "sinDelta"

== system STModel_with_MMAE/3DoF_Vehicle/Subsystem1/Pacjeka_parameters_Subsystem ==
  surface_condition : Inport  OutDataTypeStr=double  SampleTime=Ts
  Ashphalt_condition_subsystem : Subsystem  TreatAsAtomicUnit=on
  Demux : Demux  Outputs=2
  Ice_condition_subsystem : Subsystem  TreatAsAtomicUnit=on
  Merge : Merge  Inputs=4
  Snow_condition_subsystem : Subsystem  TreatAsAtomicUnit=on
  Switch Case : SwitchCase  CaseConditions={1,2,3,4}  ShowDefaultCase=off
  WetAshphalt_condition_subsystem : Subsystem  TreatAsAtomicUnit=on
  front : Outport  OutDataTypeStr=double  SampleTime=Ts
  rear : Outport  Port=2  OutDataTypeStr=double  SampleTime=Ts
  wires:
  Demux/2 -> rear/1  "rear"
  Merge/1 -> Demux/1
  Switch Case/1 -> Ashphalt_condition_subsystem/Action
  Switch Case/3 -> Snow_condition_subsystem/Action
  Demux/1 -> front/1  "front"
  surface_condition/1 -> Switch Case/1
  Ashphalt_condition_subsystem/1(Out1) -> Merge/1
  Switch Case/2 -> WetAshphalt_condition_subsystem/Action
  WetAshphalt_condition_subsystem/1(Out1) -> Merge/2
  Snow_condition_subsystem/1(Out1) -> Merge/3
  Ice_condition_subsystem/1(Out1) -> Merge/4
  Switch Case/4 -> Ice_condition_subsystem/Action

== system STModel_with_MMAE/3DoF_Vehicle/Subsystem1/Psi_ddot_subsystem ==
  cosDelta : Inport
  sinDelta : Inport  Port=2
  Fyf : Inport  Port=3
  Fyr : Inport  Port=4
  Fxf : Inport  Port=5
  psi_dot_curr : Inport  Port=6
  Add : Sum  Inputs=++-
  Add1 : Sum
  Gain : Gain  Gain=l_f
  Gain1 : Gain  Gain=l_r
  Gain2 : Gain  Gain=l_f
  Gain3 : Gain  Gain=1/Iz
  Gain4 : Gain  Gain=Tsmall
  Multiply : Product
  Multiply1 : Product
  psi_dot_next : Outport
  wires:
  cosDelta/1 -> Multiply/1
  Fyf/1 -> Multiply/2
  Multiply/1 -> Gain/1
  Fyr/1 -> Gain1/1
  sinDelta/1 -> Multiply1/1
  Fxf/1 -> Multiply1/2
  Multiply1/1 -> Gain2/1
  Gain/1 -> Add/1
  Gain2/1 -> Add/2
  Gain1/1 -> Add/3
  Add/1 -> Gain3/1  "Mz"
  Gain3/1 -> Gain4/1  "psi_ddot"
  Gain4/1 -> Add1/1
  psi_dot_curr/1 -> Add1/2
  Add1/1 -> psi_dot_next/1  "psi_dot_next"

== system STModel_with_MMAE/3DoF_Vehicle/Subsystem1/Vxdot_subsystem ==
  psi_dot_curr : Inport
  Vy_curr : Inport  Port=2
  Fxf : Inport  Port=3
  Fxr : Inport  Port=4
  Fyf : Inport  Port=5
  cosDelta : Inport  Port=6
  sinDelta : Inport  Port=7
  Vx_curr : Inport  Port=8
  Add : Sum
  Fy_subsystem : Subsystem
  Gain : Gain  Gain=1/m
  Gain1 : Gain  Gain=Ts
  Multiply : Product
  Subtract : Sum
  Vx_next : Outport
  wires:
  sinDelta/1 -> Fy_subsystem/5(sinDelta)
  cosDelta/1 -> Fy_subsystem/4(cosDelta)
  Fyf/1 -> Fy_subsystem/3(Fxr)
  Fxr/1 -> Fy_subsystem/2(Fxf)
  Fxf/1 -> Fy_subsystem/1(Fyf)
  Fy_subsystem/1(Fx) -> Gain/1
  Gain/1 -> Subtract/2
  psi_dot_curr/1 -> Multiply/1
  Vy_curr/1 -> Multiply/2
  Multiply/1 -> Subtract/1
  Subtract/1 -> Gain1/1
  Gain1/1 -> Add/1
  Vx_curr/1 -> Add/2
  Add/1 -> Vx_next/1  "Vx_next"

== system STModel_with_MMAE/3DoF_Vehicle/Subsystem1/Vydot_subsystem ==
  psi_dot_curr : Inport
  Vx_curr : Inport  Port=2
  Fyf : Inport  Port=3
  Fyr : Inport  Port=4
  Fxf : Inport  Port=5
  cosDelta : Inport  Port=6
  sinDelta : Inport  Port=7
  Vy_curr : Inport  Port=8
  Add : Sum
  Fy_subsystem : Subsystem
  Gain : Gain  Gain=1/m
  Gain1 : Gain  Gain=Ts
  Multiply : Product
  Subtract : Sum  Inputs=-+
  Vy_next : Outport
  wires:
  sinDelta/1 -> Fy_subsystem/5(sinDelta)
  cosDelta/1 -> Fy_subsystem/4(cosDelta)
  Fxf/1 -> Fy_subsystem/3(Fxf)
  Fyr/1 -> Fy_subsystem/2(Fyr)
  Fyf/1 -> Fy_subsystem/1(Fyf)
  Fy_subsystem/1(Fy) -> Gain/1
  Gain/1 -> Subtract/2
  psi_dot_curr/1 -> Multiply/1
  Vx_curr/1 -> Multiply/2
  Multiply/1 -> Subtract/1
  Subtract/1 -> Gain1/1
  Gain1/1 -> Add/1
  Vy_curr/1 -> Add/2
  Add/1 -> Vy_next/1  "Vy_next"

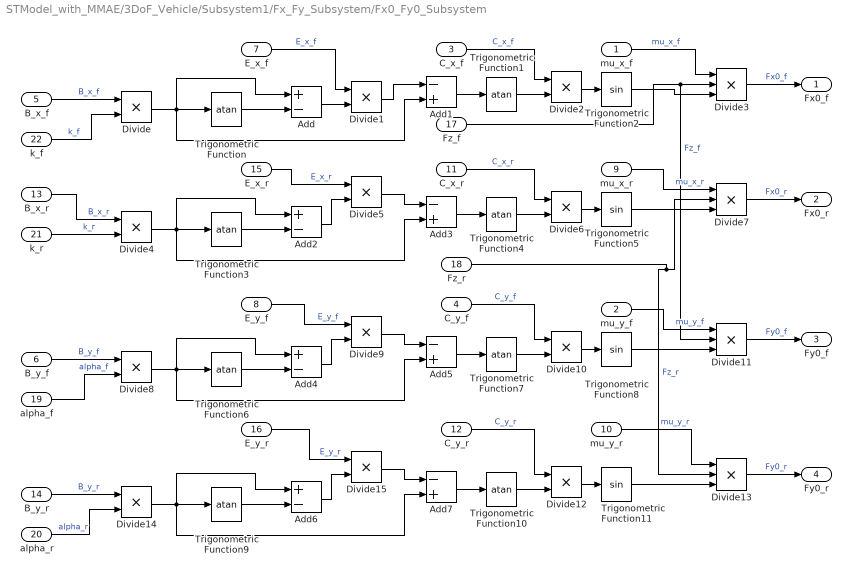
== system STModel_with_MMAE/3DoF_Vehicle/Subsystem1/Fx_Fy_Subsystem/Fx0_Fy0_Subsystem ==
  mu_x_f : Inport
  mu_y_f : Inport  Port=2
  C_x_f : Inport  Port=3
  C_y_f : Inport  Port=4
  B_x_f : Inport  Port=5
  B_y_f : Inport  Port=6
  E_x_f : Inport  Port=7
  E_y_f : Inport  Port=8
  mu_x_r : Inport  Port=9
  mu_y_r : Inport  Port=10
  C_x_r : Inport  Port=11
  C_y_r : Inport  Port=12
  B_x_r : Inport  Port=13
  B_y_r : Inport  Port=14
  E_x_r : Inport  Port=15
  E_y_r : Inport  Port=16
  Fz_f : Inport  Port=17
  Fz_r : Inport  Port=18
  alpha_f : Inport  Port=19
  alpha_r : Inport  Port=20
  k_r : Inport  Port=21
  k_f : Inport  Port=22
  Add{,2,4,6} (4 alike) : Sum  Inputs=+-
  Add{1,3,5,7} (4 alike) : Sum  Inputs=-+
  Divide{,1..2,4..6,8..10,12,14..15} (12 alike) : Product  Inputs=**
  Divide{3,7,11,13} (4 alike) : Product  Inputs=***
  Trigonometric Function{,1,3..4,6..7,9..10} (8 alike) : Trigonometry  Operator=atan
  Trigonometric Function{2,5,8,11} (4 alike) : Trigonometry
  Fx0_f : Outport
  Fx0_r : Outport  Port=2
  Fy0_f : Outport  Port=3
  Fy0_r : Outport  Port=4
  wires:
  E_y_f/1 -> Divide9/1  "E_y_f"
  B_x_f/1 -> Divide/1  "B_x_f"
  C_x_f/1 -> Divide2/1  "C_x_f"
  mu_x_f/1 -> Divide3/1  "mu_x_f"
  mu_y_f/1 -> Divide11/1  "mu_y_f"
  E_x_f/1 -> Divide1/1  "E_x_f"
  B_y_f/1 -> Divide8/1  "B_y_f"
  C_y_f/1 -> Divide10/1  "C_y_f"
  B_y_r/1 -> Divide14/1  "B_y_r"
  E_x_r/1 -> Divide5/1  "E_x_r"
  mu_x_r/1 -> Divide7/1  "mu_x_r"
  E_y_r/1 -> Divide15/1  "E_y_r"
  B_x_r/1 -> Divide4/1  "B_x_r"
  mu_y_r/1 -> Divide13/1  "mu_y_r"
  C_y_r/1 -> Divide12/1  "C_y_r"
  C_x_r/1 -> Divide6/1  "C_x_r"
  Trigonometric Function2/1 -> Divide3/3
  Divide3/1 -> Fx0_f/1  "Fx0_f"
  Divide5/1 -> Add3/1
  Trigonometric Function5/1 -> Divide7/3
  Add3/1 -> Trigonometric Function4/1
  Divide2/1 -> Trigonometric Function2/1
  Add1/1 -> Trigonometric Function1/1
  Trigonometric Function4/1 -> Divide6/2
  Divide7/1 -> Fx0_r/1  "Fx0_r"
  Add/1 -> Divide1/2
  Divide6/1 -> Trigonometric Function5/1
  Trigonometric Function3/1 -> Add2/2
  Divide/1 -> Add1/2, Add/1, Trigonometric Function/1
  Divide4/1 -> Add3/2, Add2/1, Trigonometric Function3/1
  Trigonometric Function1/1 -> Divide2/2
  Divide1/1 -> Add1/1
  Trigonometric Function/1 -> Add/2
  Add2/1 -> Divide5/2
  alpha_f/1 -> Divide8/2  "alpha_f"
  alpha_r/1 -> Divide14/2  "alpha_r"
  k_f/1 -> Divide/2  "k_f"
  k_r/1 -> Divide4/2  "k_r"
  Add4/1 -> Divide9/2
  Trigonometric Function7/1 -> Divide10/2
  Trigonometric Function6/1 -> Add4/2
  Divide10/1 -> Trigonometric Function8/1
  Divide9/1 -> Add5/1
  Fz_f/1 -> Divide11/2, Divide3/2  "Fz_f"
  Divide8/1 -> Add5/2, Add4/1, Trigonometric Function6/1
  Add5/1 -> Trigonometric Function7/1
  Trigonometric Function8/1 -> Divide11/3
  Divide11/1 -> Fy0_f/1  "Fy0_f"
  Divide13/1 -> Fy0_r/1  "Fy0_r"
  Divide14/1 -> Trigonometric Function9/1, Add7/2, Add6/1
  Fz_r/1 -> Divide13/2, Divide7/2  "Fz_r"
  Add7/1 -> Trigonometric Function10/1
  Add6/1 -> Divide15/2
  Trigonometric Function10/1 -> Divide12/2
  Divide15/1 -> Add7/1
  Trigonometric Function9/1 -> Add6/2
  Trigonometric Function11/1 -> Divide13/3
  Divide12/1 -> Trigonometric Function11/1

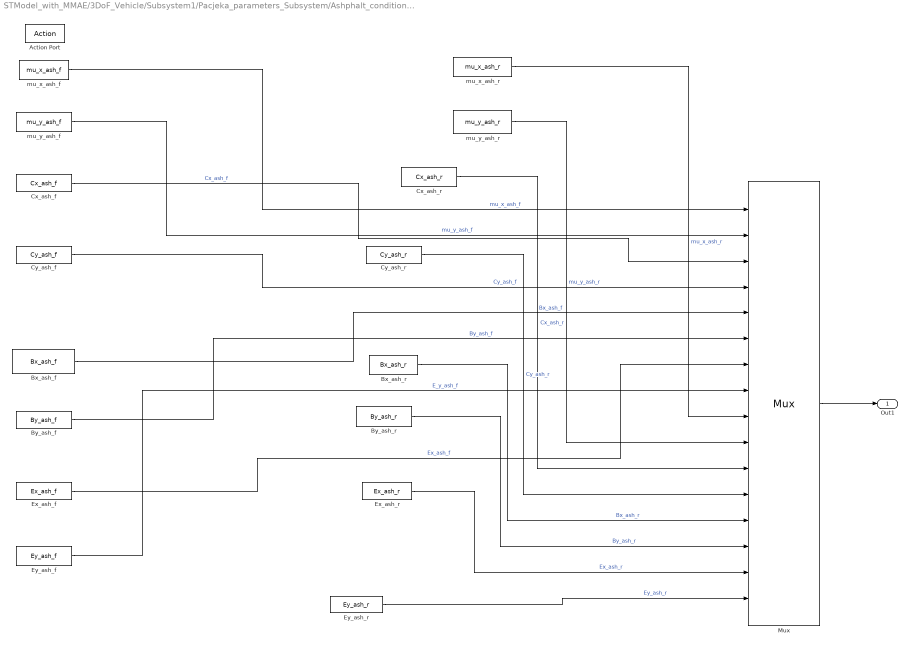
== system STModel_with_MMAE/3DoF_Vehicle/Subsystem1/Pacjeka_parameters_Subsystem/Ashphalt_condition_subsystem ==
  Action Port : ActionPort  ActionType=case
  Bx_ash_f : Constant  Value=Bx_ash_f
  Bx_ash_r : Constant  Value=Bx_ash_r
  By_ash_f : Constant  Value=By_ash_f
  By_ash_r : Constant  Value=By_ash_r
  Cx_ash_f : Constant  Value=Cx_ash_f
  Cx_ash_r : Constant  Value=Cx_ash_r
  Cy_ash_f : Constant  Value=Cy_ash_f
  Cy_ash_r : Constant  Value=Cy_ash_r
  Ex_ash_f : Constant  Value=Ex_ash_f
  Ex_ash_r : Constant  Value=Ex_ash_r
  Ey_ash_f : Constant  Value=Ey_ash_f
  Ey_ash_r : Constant  Value=Ey_ash_r
  Mux : Mux  Inputs=16
      settings: DisplayOption=signals
  mu_x_ash_f : Constant  Value=mu_x_ash_f
  mu_x_ash_r : Constant  Value=mu_x_ash_r
  mu_y_ash_f : Constant  Value=mu_y_ash_f
  mu_y_ash_r : Constant  Value=mu_y_ash_r
  Out1 : Outport  OutDataTypeStr=double  SampleTime=Ts
  wires:
  mu_x_ash_f/1 -> Mux/1  "mu_x_ash_f"
  mu_y_ash_f/1 -> Mux/2  "mu_y_ash_f"
  Cx_ash_f/1 -> Mux/3  "Cx_ash_f"
  Cy_ash_f/1 -> Mux/4  "Cy_ash_f"
  Bx_ash_f/1 -> Mux/5  "Bx_ash_f"
  By_ash_f/1 -> Mux/6  "By_ash_f"
  Ex_ash_f/1 -> Mux/7  "Ex_ash_f"
  Ey_ash_f/1 -> Mux/8  "E_y_ash_f"
  Cy_ash_r/1 -> Mux/12  "Cy_ash_r"
  Cx_ash_r/1 -> Mux/11  "Cx_ash_r"
  By_ash_r/1 -> Mux/14  "By_ash_r"
  Bx_ash_r/1 -> Mux/13  "Bx_ash_r"
  mu_y_ash_r/1 -> Mux/10  "mu_y_ash_r"
  Ex_ash_r/1 -> Mux/15  "Ex_ash_r"
  mu_x_ash_r/1 -> Mux/9  "mu_x_ash_r"
  Ey_ash_r/1 -> Mux/16  "Ey_ash_r"
  Mux/1 -> Out1/1

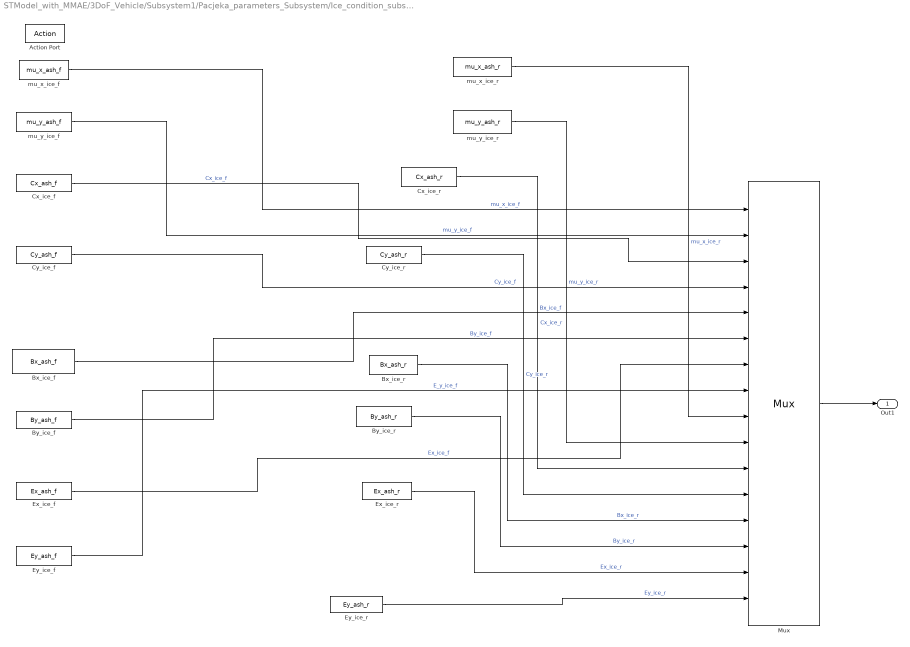
== system STModel_with_MMAE/3DoF_Vehicle/Subsystem1/Pacjeka_parameters_Subsystem/Ice_condition_subsystem ==
  Action Port : ActionPort  ActionType=case
  Bx_ice_f : Constant  Value=Bx_ash_f
  Bx_ice_r : Constant  Value=Bx_ash_r
  By_ice_f : Constant  Value=By_ash_f
  By_ice_r : Constant  Value=By_ash_r
  Cx_ice_f : Constant  Value=Cx_ash_f
  Cx_ice_r : Constant  Value=Cx_ash_r
  Cy_ice_f : Constant  Value=Cy_ash_f
  Cy_ice_r : Constant  Value=Cy_ash_r
  Ex_ice_f : Constant  Value=Ex_ash_f
  Ex_ice_r : Constant  Value=Ex_ash_r
  Ey_ice_f : Constant  Value=Ey_ash_f
  Ey_ice_r : Constant  Value=Ey_ash_r
  Mux : Mux  Inputs=16
      settings: DisplayOption=signals
  mu_x_ice_f : Constant  Value=mu_x_ash_f
  mu_x_ice_r : Constant  Value=mu_x_ash_r
  mu_y_ice_f : Constant  Value=mu_y_ash_f
  mu_y_ice_r : Constant  Value=mu_y_ash_r
  Out1 : Outport  OutDataTypeStr=double  SampleTime=Ts
  wires:
  mu_x_ice_f/1 -> Mux/1  "mu_x_ice_f"
  mu_y_ice_f/1 -> Mux/2  "mu_y_ice_f"
  Cx_ice_f/1 -> Mux/3  "Cx_ice_f"
  Cy_ice_f/1 -> Mux/4  "Cy_ice_f"
  Bx_ice_f/1 -> Mux/5  "Bx_ice_f"
  By_ice_f/1 -> Mux/6  "By_ice_f"
  Ex_ice_f/1 -> Mux/7  "Ex_ice_f"
  Ey_ice_f/1 -> Mux/8  "E_y_ice_f"
  Cy_ice_r/1 -> Mux/12  "Cy_ice_r"
  Cx_ice_r/1 -> Mux/11  "Cx_ice_r"
  By_ice_r/1 -> Mux/14  "By_ice_r"
  Bx_ice_r/1 -> Mux/13  "Bx_ice_r"
  mu_y_ice_r/1 -> Mux/10  "mu_y_ice_r"
  Ex_ice_r/1 -> Mux/15  "Ex_ice_r"
  mu_x_ice_r/1 -> Mux/9  "mu_x_ice_r"
  Ey_ice_r/1 -> Mux/16  "Ey_ice_r"
  Mux/1 -> Out1/1

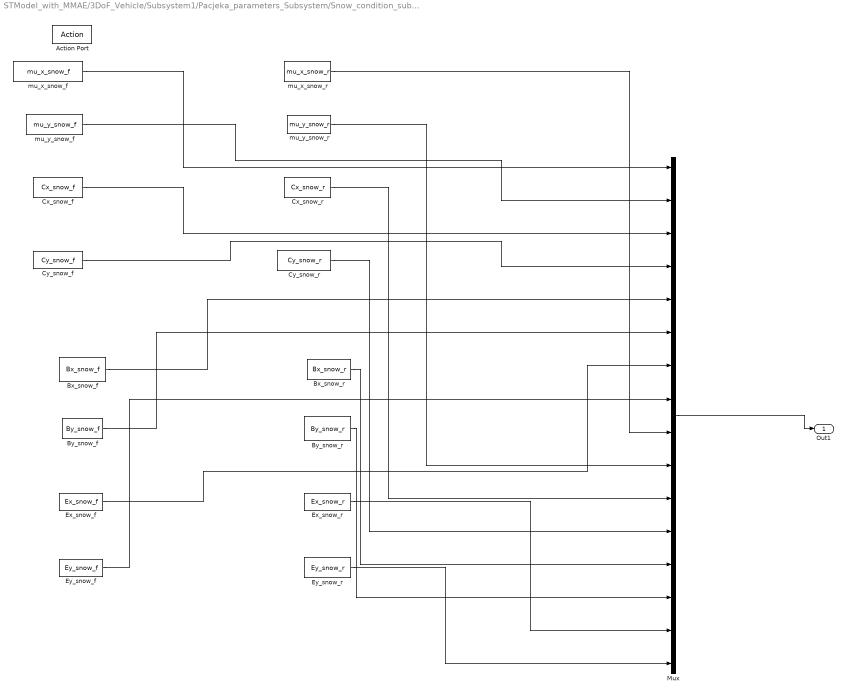
== system STModel_with_MMAE/3DoF_Vehicle/Subsystem1/Pacjeka_parameters_Subsystem/Snow_condition_subsystem ==
  Action Port : ActionPort  ActionType=case
  Bx_snow_f : Constant  Value=Bx_snow_f
  Bx_snow_r : Constant  Value=Bx_snow_r
  By_snow_f : Constant  Value=By_snow_f
  By_snow_r : Constant  Value=By_snow_r
  Cx_snow_f : Constant  Value=Cx_snow_f
  Cx_snow_r : Constant  Value=Cx_snow_r
  Cy_snow_f : Constant  Value=Cy_snow_f
  Cy_snow_r : Constant  Value=Cy_snow_r
  Ex_snow_f : Constant  Value=Ex_snow_f
  Ex_snow_r : Constant  Value=Ex_snow_r
  Ey_snow_f : Constant  Value=Ey_snow_f
  Ey_snow_r : Constant  Value=Ey_snow_r
  Mux : Mux  Inputs=16
  mu_x_snow_f : Constant  Value=mu_x_snow_f
  mu_x_snow_r : Constant  Value=mu_x_snow_r
  mu_y_snow_f : Constant  Value=mu_y_snow_f
  mu_y_snow_r : Constant  Value=mu_y_snow_r
  Out1 : Outport  OutDataTypeStr=double  SampleTime=Ts
  wires:
  Ex_snow_r/1 -> Mux/15
  Cy_snow_r/1 -> Mux/12
  By_snow_r/1 -> Mux/14
  Cx_snow_r/1 -> Mux/11
  mu_y_snow_r/1 -> Mux/10
  mu_x_snow_r/1 -> Mux/9
  Bx_snow_r/1 -> Mux/13
  Ey_snow_r/1 -> Mux/16
  mu_x_snow_f/1 -> Mux/1
  mu_y_snow_f/1 -> Mux/2
  Cx_snow_f/1 -> Mux/3
  Cy_snow_f/1 -> Mux/4
  Bx_snow_f/1 -> Mux/5
  By_snow_f/1 -> Mux/6
  Ex_snow_f/1 -> Mux/7
  Ey_snow_f/1 -> Mux/8
  Mux/1 -> Out1/1

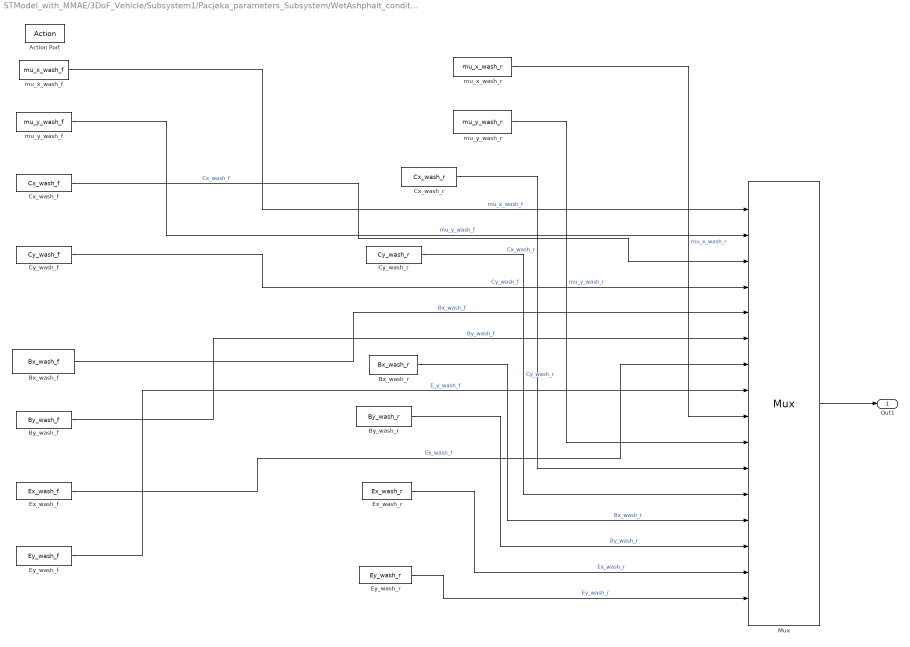
== system STModel_with_MMAE/3DoF_Vehicle/Subsystem1/Pacjeka_parameters_Subsystem/WetAshphalt_condition_subsystem ==
  Action Port : ActionPort  ActionType=case
  Bx_wash_f : Constant  Value=Bx_wash_f
  Bx_wash_r : Constant  Value=Bx_wash_r
  By_wash_f : Constant  Value=By_wash_f
  By_wash_r : Constant  Value=By_wash_r
  Cx_wash_f : Constant  Value=Cx_wash_f
  Cx_wash_r : Constant  Value=Cx_wash_r
  Cy_wash_f : Constant  Value=Cy_wash_f
  Cy_wash_r : Constant  Value=Cy_wash_r
  Ex_wash_f : Constant  Value=Ex_wash_f
  Ex_wash_r : Constant  Value=Ex_wash_r
  Ey_wash_f : Constant  Value=Ey_wash_f
  Ey_wash_r : Constant  Value=Ey_wash_r
  Mux : Mux  Inputs=16
      settings: DisplayOption=signals
  mu_x_wash_f : Constant  Value=mu_x_wash_f
  mu_x_wash_r : Constant  Value=mu_x_wash_r
  mu_y_wash_f : Constant  Value=mu_y_wash_f
  mu_y_wash_r : Constant  Value=mu_y_wash_r
  Out1 : Outport  OutDataTypeStr=double  SampleTime=Ts
  wires:
  mu_x_wash_f/1 -> Mux/1  "mu_x_wash_f"
  mu_y_wash_f/1 -> Mux/2  "mu_y_wash_f"
  Cx_wash_f/1 -> Mux/3  "Cx_wash_f"
  Cy_wash_f/1 -> Mux/4  "Cy_wash_f"
  Bx_wash_f/1 -> Mux/5  "Bx_wash_f"
  By_wash_f/1 -> Mux/6  "By_wash_f"
  Ex_wash_f/1 -> Mux/7  "Ex_wash_f"
  Ey_wash_f/1 -> Mux/8  "E_y_wash_f"
  Cy_wash_r/1 -> Mux/12  "Cy_wash_r"
  Cx_wash_r/1 -> Mux/11  "Cx_wash_r"
  By_wash_r/1 -> Mux/14  "By_wash_r"
  Bx_wash_r/1 -> Mux/13  "Bx_wash_r"
  mu_y_wash_r/1 -> Mux/10  "mu_y_wash_r"
  Ex_wash_r/1 -> Mux/15  "Ex_wash_r"
  mu_x_wash_r/1 -> Mux/9  "mu_x_wash_r"
  Ey_wash_r/1 -> Mux/16  "Ey_wash_r"
  Mux/1 -> Out1/1

== system STModel_with_MMAE/3DoF_Vehicle/Subsystem1/Vxdot_subsystem/Fy_subsystem ==
  Fyf : Inport
  Fxf : Inport  Port=2
  Fxr : Inport  Port=3
  cosDelta : Inport  Port=4
  sinDelta : Inport  Port=5
  Add : Sum  Inputs=-++
  Multiply : Product
  Multiply1 : Product
  Fx : Outport
  wires:
  Fyf/1 -> Multiply/1
  Multiply/1 -> Add/1
  Multiply1/1 -> Add/3
  Add/1 -> Fx/1
  Fxf/1 -> Multiply1/1
  cosDelta/1 -> Multiply1/2
  Fxr/1 -> Add/2
  sinDelta/1 -> Multiply/2

== system STModel_with_MMAE/3DoF_Vehicle/Subsystem1/Vydot_subsystem/Fy_subsystem ==
  Fyf : Inport
  Fyr : Inport  Port=2
  Fxf : Inport  Port=3
  cosDelta : Inport  Port=4
  sinDelta : Inport  Port=5
  Add : Sum  Inputs=3
  Multiply : Product
  Multiply1 : Product
  Fy : Outport
  wires:
  Fyf/1 -> Multiply/1
  cosDelta/1 -> Multiply/2
  Multiply/1 -> Add/1
  Fyr/1 -> Add/2
  Fxf/1 -> Multiply1/1
  sinDelta/1 -> Multiply1/2
  Multiply1/1 -> Add/3
  Add/1 -> Fy/1

== matlab function STModel_with_MMAE/Behavior Identification/EKF for right Lane Change/MATLAB Function1 ==
  data: X input; P input; u input; X_hat_plus output; y_tilde input; P_plus output; ek_minus output; ek_m_covariance output; wk output; p_yk_xkminus output; wk_prev input; maneuver_length input
function [X_hat_plus, P_plus, ek_minus, ek_m_covariance, wk, p_yk_xkminus] = EKFRightLaneChangeCustom(X, P, u, y_tilde, wk_prev, maneuver_length)

    %%
    %TODO: See how can this be moved out of the function later
    %sampling time
    Ts_bp = 0.01;
%     maneuver_length = 150;  %m
    lane_center_to_center_distance = 3.5;   %meters

    % measurement noise covariance
%     R = [0.2 0; 0 0.2];
    R = [0.025 0; 0 0.025];
    
    % process noise covariance
%     Q = diag([0.5 5.0 0.5 5.0]);
    Q = diag([0.005 0.005 0.005 0.005]);

    % states - X = [x vx y vy] -     
    Ck = [1 0 0 0; 0 0 1 0];

    F = rightLaneChangeParametricJacobianFcn(X, u, maneuver_length, lane_center_to_center_distance);
    %%
    % Now estimate states using kalman filter
    
    %predict
    xhat_minus = rightLaneChangeParametricFcn(X, u, maneuver_length, lane_center_to_center_distance);
    P_minus = (F * P * F') + Ts_bp*Q;
    yhat_minus = Ck * xhat_minus;

    %correct
    ek_minus = y_tilde - yhat_minus;    %residual
    ek_m_covariance = Ck * P_minus *Ck' + R;    %residual covariance
    K = P_minus * Ck' * inv(ek_m_covariance);
    X_hat_plus = xhat_minus + K * ek_minus;
    P_plus = (eye(4) - K * Ck) * P_minus;

    %calculate MMAE weights
    p_yk_xkminus = 1/sqrt(det(2*pi*ek_m_covariance))*exp(-1/2 * ek_minus'* inv(ek_m_covariance) * ek_minus);
    wk = wk_prev * p_yk_xkminus;

end
